simulink model "IEEE13bus_v2019b_Discrete_PI_ZIPload"  (R2024a)
settings: Solver=ode4  StartTime=0.0  StopTime=5  FixedStep=Ts  MaxStep=1e-4  RelTol=1e-4
InitFcn:
  | a=1; % Loading Factor
  | Ts=50e-6;
  | % phase to sequence conversion of RXB matrices
  | c=1*exp(sqrt(-1)*(120*pi/180));
  | T=[1 1 1;1 c*c c;1 c c*c];
  | Tinv=1/3*[1 1 1;1 c c*c;1 c*c c];
  | 
  | % Simulation data for the IEEE 13 Node Test Feeder model
  | mi2km = 1.60934;%  miles to km conversion
  | ft2km = 0.0003048; % feet to km conversion
  | ms2F = 1*1e-6/(2*pi*60);% microsiemens to Farads conversion
  | 
  | 
  | %% Configuration 601
  | % Series Resitance and Reactance - ohm/mile
  | R_601 = [0.3465 0.1560 0.1580;0.1560 0.3375 0.1535;0.1580 0.1535 0.3414];
  | X_601 = [1.1079 0.5017 0.4236;0.5017 1.0478 0.3849;0.4236 0.3849 1.0348];
  | % charging susceptance - microsiemens/mile
  | B_601 = [6.2998 -1.9958 -1.2595;-1.9958 5.9597 -0.7417;-1.2595 -0.7417 5.6386];
  | 
  | R_601 = R_601/mi2km;
  | Rseq=Tinv*R_601*T;
  | R1_601=Rseq(2,2);R0_601=Rseq(1,1);
  | 
  | L_601 = (X_601/(2*pi*60))/mi2km;
  | Lseq=Tinv*L_601*T;
  | L1_601=Lseq(2,2);L0_601=Lseq(1,1);
  | 
  | C_601 =(B_601*ms2F)/mi2km;
  | Cseq=Tinv*C_601*T;
  | C1_601=Cseq(2,2);C0_601=Cseq(1,1);
  | 
  | %% Configuration 602 - series reactance - ohm/mile
  | R_602 = [0.7526 0.1580 0.1560;0.1580 0.7475 0.1535;0.1560 0.1535 0.7436];
  | X_602 = [1.1814 0.4236 0.5017;0.4236 1.1983 0.3849;0.5017 0.3849 1.2112];
  | % charging susceptance - microsiemens/mile
  | B_602 = [5.6990 -1.0817 -1.6905;-1.0817 5.1795 -0.6588;-1.6905 -0.6588 5.4246];
  | 
  | R_602 = R_602/mi2km;
  | Rseq=Tinv*R_602*T;
  | R1_602=Rseq(2,2);R0_602=Rseq(1,1);
  | 
  | L_602 = (X_602/(2*pi*60))/mi2km;
  | Lseq=Tinv*L_602*T;
  | L1_602=Lseq(2,2);L0_602=Lseq(1,1);
  | 
  | C_602 =(B_602*ms2F)/mi2km;
  | Cseq=Tinv*C_602*T;
  | C1_602=Cseq(2,2);C0_602=Cseq(1,1);
  | %% Configuration 603 - series reactance - ohm/mile
  | R_603 = [0 0 0;0 1.3294 0.2066;0 0.2066 1.3238];
  | X_603 = [0 0 0;0 1.3471 0.4591;0 0.4591 1.3569];
  | % charging susceptance - microsiemens/mile
  | B_603 = [0 0 0;0 4.7097 -0.8999;0 -0.8999 4.6658];
  | 
  | % convert for SPS
  | R_603 = R_603/mi2km;
  | Rseq=Tinv*R_603*T;
  | R1_603=Rseq(2,2);R0_603=Rseq(1,1);
  | 
  | ... (+71 lines)
undefined symbols (not defined in the file or in its folder): find_system
libraries: spsSeriesRLCBranchLib x61, spsGroundLib x52, spsFourierLib x30, spsControlledCurrentSourceLib x28, spsVoltageMeasurementLib x28, spsThreePhaseVIMeasurementLib x16, spsOnDelayLib x6, spsThreePhasePISectionLineLib x5, spsMutualInductanceLib x4, spsRMSLib x4, spsParallelRLCBranchLib x3, spsLinearTransformerLib x3
(part 4 of 4)

== system IEEE13bus_v2019b_Discrete_PI_ZIPload/Regulator 1/Single Phase SVR_A/Voltage Regulator Control/Tap Changer Control/Edge Detector/NEGATIVE Edge ==
  IN : Inport
  IN previous : Inport  Port=2
  Enable : EnablePort  PropagateVarSize=During execution
  Relational Operator1 : RelationalOperator  Operator=>
  OUT : Outport  VectorParamsAs1DForOutWhenUnconnected=off
  wires:
  Relational Operator1/1 -> OUT/1
  IN previous/1 -> Relational Operator1/1
  IN/1 -> Relational Operator1/2

== system IEEE13bus_v2019b_Discrete_PI_ZIPload/Regulator 1/Single Phase SVR_A/Voltage Regulator Control/Tap Changer Control/Edge Detector/POSITIVE Edge ==
  IN : Inport
  IN previous : Inport  Port=2
  Enable : EnablePort  PropagateVarSize=During execution
  Relational Operator1 : RelationalOperator  Operator=>
  OUT : Outport  VectorParamsAs1DForOutWhenUnconnected=off
  wires:
  Relational Operator1/1 -> OUT/1
  IN previous/1 -> Relational Operator1/2
  IN/1 -> Relational Operator1/1

== system IEEE13bus_v2019b_Discrete_PI_ZIPload/Regulator 1/Single Phase SVR_B/Voltage Regulator Control/Tap Changer Control/Edge Detector/NEGATIVE Edge ==
  IN : Inport
  IN previous : Inport  Port=2
  Enable : EnablePort  PropagateVarSize=During execution
  Relational Operator1 : RelationalOperator  Operator=>
  OUT : Outport  VectorParamsAs1DForOutWhenUnconnected=off
  wires:
  IN/1 -> Relational Operator1/2
  IN previous/1 -> Relational Operator1/1
  Relational Operator1/1 -> OUT/1

== system IEEE13bus_v2019b_Discrete_PI_ZIPload/Regulator 1/Single Phase SVR_B/Voltage Regulator Control/Tap Changer Control/Edge Detector/POSITIVE Edge ==
  IN : Inport
  IN previous : Inport  Port=2
  Enable : EnablePort  PropagateVarSize=During execution
  Relational Operator1 : RelationalOperator  Operator=>
  OUT : Outport  VectorParamsAs1DForOutWhenUnconnected=off
  wires:
  IN/1 -> Relational Operator1/1
  IN previous/1 -> Relational Operator1/2
  Relational Operator1/1 -> OUT/1

== system IEEE13bus_v2019b_Discrete_PI_ZIPload/Regulator 1/Single Phase SVR_C/Voltage Regulator Control/Tap Changer Control/Edge Detector/NEGATIVE Edge ==
  IN : Inport
  IN previous : Inport  Port=2
  Enable : EnablePort  PropagateVarSize=During execution
  Relational Operator1 : RelationalOperator  Operator=>
  OUT : Outport  VectorParamsAs1DForOutWhenUnconnected=off
  wires:
  Relational Operator1/1 -> OUT/1
  IN previous/1 -> Relational Operator1/1
  IN/1 -> Relational Operator1/2

== system IEEE13bus_v2019b_Discrete_PI_ZIPload/Regulator 1/Single Phase SVR_C/Voltage Regulator Control/Tap Changer Control/Edge Detector/POSITIVE Edge ==
  IN : Inport
  IN previous : Inport  Port=2
  Enable : EnablePort  PropagateVarSize=During execution
  Relational Operator1 : RelationalOperator  Operator=>
  OUT : Outport  VectorParamsAs1DForOutWhenUnconnected=off
  wires:
  Relational Operator1/1 -> OUT/1
  IN previous/1 -> Relational Operator1/2
  IN/1 -> Relational Operator1/1

== matlab function IEEE13bus_v2019b_Discrete_PI_ZIPload/634 Yg PQ/Embedded MATLAB Function1 ==
  data: Iinjinst output; Vmeas input; LoadType parameter; Vnom parameter; Pnom parameter; Qnom parameter; Vlim parameter; fnom parameter; clock input; Ddel input
%Three Phase Star ZIP Load
%Author: Arun Suresh, University of North Carolina, Charlotte
%Pl=Pnom(Kz*(Vmeas/Vnom)^2+Ki(Vmeas/Vnom)+Kp), nom-nominal value,meas-measured value
%Ql=Qnom(Kz*(Vmeas/Vnom)^2+Ki(Vmeas/Vnom)+Kp), nom-nominal value,meas-measured value
%Iinj=((Pl+jQl)/Vmeas)'
function Iinjinst  = InjectedCurrent(Vmeas,LoadType,Vnom,Pnom,Qnom,Vlim,fnom,clock,Ddel)
% Calculate Pl and Ql.
Kz=0;Ki=0;Kp=0;
Vk=abs(Vmeas/(Vnom/sqrt(3)));%(Vmeas/Vnom)
switch LoadType  % 1 for Constant Z, 2 for Constant I and 3 for Constant P, 
    case 1
        Kz=1;
    case 2
        if Vk >= Vlim % convert to Constant Z load due to voltage violation
            Ki=1;
        else
            Kz=1;
        end
    case 3
        if Vk >= Vlim % convert to Constant Z load due to voltage violation
           Kp=1;
        else
            Kz=1;
        end          
 
end
Pl=Pnom'.*((Kz*Vk.*Vk)+(Ki*Vk)+(Kp));
Ql=Qnom'.*((Kz*Vk.*Vk)+(Ki*Vk)+(Kp));
% Net Injected Curent.
% j=sqrt(-1);
Iinj = conj((Pl+j*Ql)./Vmeas);
Iinjinsta =abs(Iinj(1))*sqrt(2)*sin(2*fnom*pi*clock + angle(Iinj(1))+Ddel(1));
Iinjinstb =abs(Iinj(2))*sqrt(2)*sin(2*fnom*pi*clock + angle(Iinj(2))+Ddel(2));
Iinjinstc =abs(Iinj(3))*sqrt(2)*sin(2*fnom*pi*clock + angle(Iinj(3))+Ddel(3));
Iinjinst=[Iinjinsta  Iinjinstb  Iinjinstc]';

== matlab function IEEE13bus_v2019b_Discrete_PI_ZIPload/675 Y PQ/Embedded MATLAB Function1 ==
  data: Iinjinst output; Vmeas input; LoadType parameter; Vnom parameter; Pnom parameter; Qnom parameter; Vlim parameter; fnom parameter; clock input; Ddel input
%Three Phase Star ZIP Load
%Author: Arun Suresh, University of North Carolina, Charlotte
%Pl=Pnom(Kz*(Vmeas/Vnom)^2+Ki(Vmeas/Vnom)+Kp), nom-nominal value,meas-measured value
%Ql=Qnom(Kz*(Vmeas/Vnom)^2+Ki(Vmeas/Vnom)+Kp), nom-nominal value,meas-measured value
%Iinj=((Pl+jQl)/Vmeas)'
function Iinjinst  = InjectedCurrent(Vmeas,LoadType,Vnom,Pnom,Qnom,Vlim,fnom,clock,Ddel)
% Calculate Pl and Ql.
Kz=0;Ki=0;Kp=0;
Vk=abs(Vmeas/(Vnom/sqrt(3)));%(Vmeas/Vnom)
switch LoadType  % 1 for Constant Z, 2 for Constant I and 3 for Constant P, 
    case 1
        Kz=1;
    case 2
        if Vk >= Vlim % convert to Constant Z load due to voltage violation
            Ki=1;
        else
            Kz=1;
        end
    case 3
        if Vk >= Vlim % convert to Constant Z load due to voltage violation
           Kp=1;
        else
            Kz=1;
        end          
 
end
Pl=Pnom'.*((Kz*Vk.*Vk)+(Ki*Vk)+(Kp));
Ql=Qnom'.*((Kz*Vk.*Vk)+(Ki*Vk)+(Kp));
% Net Injected Curent.
% j=sqrt(-1);
Iinj = conj((Pl+j*Ql)./Vmeas);
Iinjinsta =abs(Iinj(1))*sqrt(2)*sin(2*fnom*pi*clock + angle(Iinj(1))+Ddel(1));
Iinjinstb =abs(Iinj(2))*sqrt(2)*sin(2*fnom*pi*clock + angle(Iinj(2))+Ddel(2));
Iinjinstc =abs(Iinj(3))*sqrt(2)*sin(2*fnom*pi*clock + angle(Iinj(3))+Ddel(3));
Iinjinst=[Iinjinsta  Iinjinstb  Iinjinstc]';

== matlab function IEEE13bus_v2019b_Discrete_PI_ZIPload/671 Yg PQ/Embedded MATLAB Function1 ==
  data: Iinjinst output; Vmeas input; LoadType parameter; Vnom parameter; Pnom parameter; Qnom parameter; Vlim parameter; fnom parameter; clock input; Ddel input
%Three Phase Star ZIP Load
%Author: Arun Suresh, University of North Carolina, Charlotte
%Pl=Pnom(Kz*(Vmeas/Vnom)^2+Ki(Vmeas/Vnom)+Kp), nom-nominal value,meas-measured value
%Ql=Qnom(Kz*(Vmeas/Vnom)^2+Ki(Vmeas/Vnom)+Kp), nom-nominal value,meas-measured value
%Iinj=((Pl+jQl)/Vmeas)'
function Iinjinst  = InjectedCurrent(Vmeas,LoadType,Vnom,Pnom,Qnom,Vlim,fnom,clock,Ddel)
% Calculate Pl and Ql.
Kz=0;Ki=0;Kp=0;
Vk=abs(Vmeas/(Vnom/sqrt(3)));%(Vmeas/Vnom)
switch LoadType  % 1 for Constant Z, 2 for Constant I and 3 for Constant P, 
    case 1
        Kz=1;
    case 2
        if Vk >= Vlim % convert to Constant Z load due to voltage violation
            Ki=1;
        else
            Kz=1;
        end
    case 3
        if Vk >= Vlim % convert to Constant Z load due to voltage violation
           Kp=1;
        else
            Kz=1;
        end          
 
end
Pl=Pnom'.*((Kz*Vk.*Vk)+(Ki*Vk)+(Kp));
Ql=Qnom'.*((Kz*Vk.*Vk)+(Ki*Vk)+(Kp));
% Net Injected Curent.
% j=sqrt(-1);
Iinj = conj((Pl+j*Ql)./Vmeas);
Iinjinsta =abs(Iinj(1))*sqrt(2)*sin(2*fnom*pi*clock + angle(Iinj(1))+Ddel(1));
Iinjinstb =abs(Iinj(2))*sqrt(2)*sin(2*fnom*pi*clock + angle(Iinj(2))+Ddel(2));
Iinjinstc =abs(Iinj(3))*sqrt(2)*sin(2*fnom*pi*clock + angle(Iinj(3))+Ddel(3));
Iinjinst=[Iinjinsta  Iinjinstb  Iinjinstc]';

== matlab function IEEE13bus_v2019b_Discrete_PI_ZIPload/671 D PQ/Embedded MATLAB Function1 ==
  data: Iinjinst output; Vmeas input; LoadType parameter; Vnom parameter; Pnom parameter; Qnom parameter; Vlim parameter; fnom parameter; clock input; Ddel input
%Three Phase Delta ZIP Load
%Author: Arun Suresh, University of North Carolina, Charlotte
%Pl=Pnom(Kz*(Vmeas/Vnom)^2+Ki(Vmeas/Vnom)+Kp), nom-nominal value,meas-measured value
%Ql=Qnom(Kz*(Vmeas/Vnom)^2+Ki(Vmeas/Vnom)+Kp), nom-nominal value,meas-measured value
%Iinj=((Pl+jQl)/Vmeas)'
function Iinjinst  = InjectedCurrent(Vmeas,LoadType,Vnom,Pnom,Qnom,Vlim,fnom,clock,Ddel)
% Calculate Pl and Ql.
Kz=0;Ki=0;Kp=0;
Vk=abs(Vmeas/(Vnom));%(Vmeas/Vnom)
switch LoadType  % 1 for Constant Z, 2 for Constant I and 3 for Constant P, 
    case 1
        Kz=1;
    case 2
        if Vk >= Vlim % convert to Constant Z load due to voltage violation
            Ki=1;
        else
            Kz=1;
        end
    case 3
        if Vk >= Vlim % convert to Constant Z load due to voltage violation
           Kp=1;
        else
            Kz=1;
        end          
 
end
Pl=Pnom'.*((Kz*Vk.*Vk)+(Ki*Vk)+(Kp));
Ql=Qnom'.*((Kz*Vk.*Vk)+(Ki*Vk)+(Kp));
% Net Injected Curent.
% j=sqrt(-1);
Iinj = conj((Pl+j*Ql)./Vmeas);
Iinjinsta =abs(Iinj(1))*sqrt(2)*sin(2*fnom*pi*clock + angle(Iinj(1))+Ddel(1));
Iinjinstb =abs(Iinj(2))*sqrt(2)*sin(2*fnom*pi*clock + angle(Iinj(2))+Ddel(2));
Iinjinstc =abs(Iinj(3))*sqrt(2)*sin(2*fnom*pi*clock + angle(Iinj(3))+Ddel(3));
Iinjinst=[Iinjinsta  Iinjinstb  Iinjinstc]';

== matlab function IEEE13bus_v2019b_Discrete_PI_ZIPload/632 Yg PQ/Embedded MATLAB Function1 ==
  data: Iinjinst output; Vmeas input; LoadType parameter; Vnom parameter; Pnom parameter; Qnom parameter; Vlim parameter; fnom parameter; clock input; Ddel input
%Three Phase Star ZIP Load
%Author: Arun Suresh, University of North Carolina, Charlotte
%Pl=Pnom(Kz*(Vmeas/Vnom)^2+Ki(Vmeas/Vnom)+Kp), nom-nominal value,meas-measured value
%Ql=Qnom(Kz*(Vmeas/Vnom)^2+Ki(Vmeas/Vnom)+Kp), nom-nominal value,meas-measured value
%Iinj=((Pl+jQl)/Vmeas)'
function Iinjinst  = InjectedCurrent(Vmeas,LoadType,Vnom,Pnom,Qnom,Vlim,fnom,clock,Ddel)
% Calculate Pl and Ql.
Kz=0;Ki=0;Kp=0;
Vk=abs(Vmeas/(Vnom/sqrt(3)));%(Vmeas/Vnom)
switch LoadType  % 1 for Constant Z, 2 for Constant I and 3 for Constant P, 
    case 1
        Kz=1;
    case 2
        if Vk >= Vlim % convert to Constant Z load due to voltage violation
            Ki=1;
        else
            Kz=1;
        end
    case 3
        if Vk >= Vlim % convert to Constant Z load due to voltage violation
           Kp=1;
        else
            Kz=1;
        end          
 
end
Pl=Pnom'.*((Kz*Vk.*Vk)+(Ki*Vk)+(Kp));
Ql=Qnom'.*((Kz*Vk.*Vk)+(Ki*Vk)+(Kp));
% Net Injected Curent.
% j=sqrt(-1);
Iinj = conj((Pl+j*Ql)./Vmeas);
Iinjinsta =abs(Iinj(1))*sqrt(2)*sin(2*fnom*pi*clock + angle(Iinj(1))+Ddel(1));
Iinjinstb =abs(Iinj(2))*sqrt(2)*sin(2*fnom*pi*clock + angle(Iinj(2))+Ddel(2));
Iinjinstc =abs(Iinj(3))*sqrt(2)*sin(2*fnom*pi*clock + angle(Iinj(3))+Ddel(3));
Iinjinst=[Iinjinsta  Iinjinstb  Iinjinstc]';

== matlab function IEEE13bus_v2019b_Discrete_PI_ZIPload/645Y PQ/Embedded MATLAB Function ==
  data: Iinjinst output; Vmeas input; LoadType parameter; Vnom parameter; Pnom parameter; Qnom parameter; Vlim parameter; fnom parameter; clock input; Ddel input
%Single Phase ZIP Load
%Author: Arun Suresh, University of North Carolina, Charlotte
%Iinj=((Pnom+jQnom)/Vmeas)'
function Iinjinst = InjectedCurrent(Vmeas,LoadType,Vnom,Pnom,Qnom,Vlim,fnom,clock,Ddel)
% Calculate Pl and Ql.
%  Vmeas=1.2303e+03 + 1.9328e+03i;
Kz=0;Ki=0;Kp=0;
Vk=(abs(Vmeas)/Vnom);%(Vmeas/Vnom)
switch LoadType  % 1 for Constant Z, 2 for Constant I and 3 for Constant P, 
    case 1
        Kz=1;
    case 2
        if Vk >= Vlim % convert to Constant Z load due to voltage violation
            Ki=1;
        else
            Kz=1;
        end
    case 3
        if Vk >= Vlim % convert to Constant Z load due to voltage violation
           Kp=1;
        else
            Kz=1;
        end          
 
end
Pl=Pnom *((Kz*Vk*Vk)+(Ki*Vk)+(Kp));
Ql=Qnom *((Kz*Vk*Vk)+(Ki*Vk)+(Kp));
% Net Injected Curent.
% j=sqrt(-1);
Iinj = conj((Pl+j*Ql)/Vmeas);
Iinjinst =abs(Iinj)*sqrt(2)*sin(2*fnom*pi*clock + angle(Iinj)+Ddel);
yt=Iinj;

== matlab function IEEE13bus_v2019b_Discrete_PI_ZIPload/646 Z/Embedded MATLAB Function ==
  data: Iinjinst output; Vmeas input; LoadType parameter; Vnom parameter; Pnom parameter; Qnom parameter; Vlim parameter; fnom parameter; clock input; Ddel input
%Single Phase ZIP Load
%Author: Arun Suresh, University of North Carolina, Charlotte
%Iinj=((Pnom+jQnom)/Vmeas)'
function Iinjinst = InjectedCurrent(Vmeas,LoadType,Vnom,Pnom,Qnom,Vlim,fnom,clock,Ddel)
% Calculate Pl and Ql.
%  Vmeas=1.2303e+03 + 1.9328e+03i;
Kz=0;Ki=0;Kp=0;
Vk=(abs(Vmeas)/Vnom);%(Vmeas/Vnom)
switch LoadType  % 1 for Constant Z, 2 for Constant I and 3 for Constant P, 
    case 1
        Kz=1;
    case 2
        if Vk >= Vlim % convert to Constant Z load due to voltage violation
            Ki=1;
        else
            Kz=1;
        end
    case 3
        if Vk >= Vlim % convert to Constant Z load due to voltage violation
           Kp=1;
        else
            Kz=1;
        end          
 
end
Pl=Pnom *((Kz*Vk*Vk)+(Ki*Vk)+(Kp));
Ql=Qnom *((Kz*Vk*Vk)+(Ki*Vk)+(Kp));
% Net Injected Curent.
% j=sqrt(-1);
Iinj = conj((Pl+j*Ql)/Vmeas);
Iinjinst =abs(Iinj)*sqrt(2)*sin(2*fnom*pi*clock + angle(Iinj)+Ddel);
yt=Iinj;

== matlab function IEEE13bus_v2019b_Discrete_PI_ZIPload/611Y I/Embedded MATLAB Function ==
  data: Iinjinst output; Vmeas input; LoadType parameter; Vnom parameter; Pnom parameter; Qnom parameter; Vlim parameter; fnom parameter; clock input; Ddel input
%Single Phase ZIP Load
%Author: Arun Suresh, University of North Carolina, Charlotte
%Iinj=((Pnom+jQnom)/Vmeas)'
function Iinjinst = InjectedCurrent(Vmeas,LoadType,Vnom,Pnom,Qnom,Vlim,fnom,clock,Ddel)
% Calculate Pl and Ql.
%  Vmeas=1.2303e+03 + 1.9328e+03i;
Kz=0;Ki=0;Kp=0;
Vk=(abs(Vmeas)/Vnom);%(Vmeas/Vnom)
switch LoadType  % 1 for Constant Z, 2 for Constant I and 3 for Constant P, 
    case 1
        Kz=1;
    case 2
        if Vk >= Vlim % convert to Constant Z load due to voltage violation
            Ki=1;
        else
            Kz=1;
        end
    case 3
        if Vk >= Vlim % convert to Constant Z load due to voltage violation
           Kp=1;
        else
            Kz=1;
        end          
 
end
Pl=Pnom *((Kz*Vk*Vk)+(Ki*Vk)+(Kp));
Ql=Qnom *((Kz*Vk*Vk)+(Ki*Vk)+(Kp));
% Net Injected Curent.
% j=sqrt(-1);
Iinj = conj((Pl+j*Ql)/Vmeas);
Iinjinst =abs(Iinj)*sqrt(2)*sin(2*fnom*pi*clock + angle(Iinj)+Ddel);
yt=Iinj;

== matlab function IEEE13bus_v2019b_Discrete_PI_ZIPload/652Y Z/Embedded MATLAB Function ==
  data: Iinjinst output; Vmeas input; LoadType parameter; Vnom parameter; Pnom parameter; Qnom parameter; Vlim parameter; fnom parameter; clock input; Ddel input
%Single Phase ZIP Load
%Author: Arun Suresh, University of North Carolina, Charlotte
%Iinj=((Pnom+jQnom)/Vmeas)'
function Iinjinst = InjectedCurrent(Vmeas,LoadType,Vnom,Pnom,Qnom,Vlim,fnom,clock,Ddel)
% Calculate Pl and Ql.
%  Vmeas=1.2303e+03 + 1.9328e+03i;
Kz=0;Ki=0;Kp=0;
Vk=(abs(Vmeas)/Vnom);%(Vmeas/Vnom)
switch LoadType  % 1 for Constant Z, 2 for Constant I and 3 for Constant P, 
    case 1
        Kz=1;
    case 2
        if Vk >= Vlim % convert to Constant Z load due to voltage violation
            Ki=1;
        else
            Kz=1;
        end
    case 3
        if Vk >= Vlim % convert to Constant Z load due to voltage violation
           Kp=1;
        else
            Kz=1;
        end          
 
end
Pl=Pnom *((Kz*Vk*Vk)+(Ki*Vk)+(Kp));
Ql=Qnom *((Kz*Vk*Vk)+(Ki*Vk)+(Kp));
% Net Injected Curent.
% j=sqrt(-1);
Iinj = conj((Pl+j*Ql)/Vmeas);
Iinjinst =abs(Iinj)*sqrt(2)*sin(2*fnom*pi*clock + angle(Iinj)+Ddel);
yt=Iinj;

== matlab function IEEE13bus_v2019b_Discrete_PI_ZIPload/692 D I/Embedded MATLAB Function1 ==
  data: Iinjinst output; Vmeas input; LoadType parameter; Vnom parameter; Pnom parameter; Qnom parameter; Vlim parameter; fnom parameter; clock input; Ddel input
%Three Phase Delta ZIP Load
%Author: Arun Suresh, University of North Carolina, Charlotte
%Pl=Pnom(Kz*(Vmeas/Vnom)^2+Ki(Vmeas/Vnom)+Kp), nom-nominal value,meas-measured value
%Ql=Qnom(Kz*(Vmeas/Vnom)^2+Ki(Vmeas/Vnom)+Kp), nom-nominal value,meas-measured value
%Iinj=((Pl+jQl)/Vmeas)'
function Iinjinst  = InjectedCurrent(Vmeas,LoadType,Vnom,Pnom,Qnom,Vlim,fnom,clock,Ddel)
% Calculate Pl and Ql.
Kz=0;Ki=0;Kp=0;
Vk=abs(Vmeas/(Vnom));%(Vmeas/Vnom)
switch LoadType  % 1 for Constant Z, 2 for Constant I and 3 for Constant P, 
    case 1
        Kz=1;
    case 2
        if Vk >= Vlim % convert to Constant Z load due to voltage violation
            Ki=1;
        else
            Kz=1;
        end
    case 3
        if Vk >= Vlim % convert to Constant Z load due to voltage violation
           Kp=1;
        else
            Kz=1;
        end          
 
end
Pl=Pnom'.*((Kz*Vk.*Vk)+(Ki*Vk)+(Kp));
Ql=Qnom'.*((Kz*Vk.*Vk)+(Ki*Vk)+(Kp));
% Net Injected Curent.
% j=sqrt(-1);
Iinj = conj((Pl+j*Ql)./Vmeas);
Iinjinsta =abs(Iinj(1))*sqrt(2)*sin(2*fnom*pi*clock + angle(Iinj(1))+Ddel(1));
Iinjinstb =abs(Iinj(2))*sqrt(2)*sin(2*fnom*pi*clock + angle(Iinj(2))+Ddel(2));
Iinjinstc =abs(Iinj(3))*sqrt(2)*sin(2*fnom*pi*clock + angle(Iinj(3))+Ddel(3));
Iinjinst=[Iinjinsta  Iinjinstb  Iinjinstc]';
